simulink model "sim_validation_6DoFDQG_3DoF_fullq"  (R2024b)
settings: Solver=VariableStepAuto  StartTime=0.0  StopTime=tf  RelTol=1e-12  AbsTol=1e-12
values from neighbouring files (symbols this model uses):
  alpha = 0.5086    [3DoF_deterministic_Workspace.mat]    (also in Compressed_Time_Step_2dof_Experiment.mat; Copy_of_Deterministic_6DoF.m; Copy_of_Deterministic_6DoF_quat.m; Copy_of_SCP_Earth_Mars_transfer_GA_uniform_adaptive.m = 1)
  I = 0.15    [3DoF_deterministic_Workspace.mat]    (also in Copy_of_DQG_6DoF_fixedtf.m = [4.2; 4.2; 0.6]; Copy_of_Deterministic_6DoF.m = [50000; 150000; 150000] * (1e-3) ^ 2; Copy_of_Deterministic_6DoF_quat.m = [50000; 150000; 150000] * (1e-3) ^ 2; DQG_6DoF.m = [4.2; 4.2; 0.6])
  input_vector = 1:nu    [Deterministic_3DoF_with_mass_convexified_reynolds.m]    (also in Deterministic_3DoF_with_mass_convexified_takeoffdivert.m; Deterministic_3DoF_with_mass_polar.m; Deterministic_6DoF.m; Deterministic_6DoF_reynolds.m)
  L = 0.003    [3DoF_deterministic_Workspace.mat]    (also in Compressed_Time_Step_2dof_Experiment.mat; Copy_of_DQG_6DoF_fixedtf.m = 1; Copy_of_Deterministic_6DoF.m; Copy_of_Deterministic_6DoF_quat.m)
  m_0 = 2100    [3DoF_deterministic_Workspace.mat]    (also in Compressed_Time_Step_2dof_Experiment.mat = 2000; Copy_of_Deterministic_6DoF.m = 2600; Copy_of_Deterministic_6DoF_quat.m = 2600; Copy_of_SCP_Earth_Mars_transfer_GA_uniform_adaptive.m = 1)
  r_0_6DoF = [r_0(1); 0; r_0(2)]    [Deterministic_3DoF_with_mass_convexified_reynolds.m]    (also in Deterministic_3DoF_with_mass_convexified_takeoffdivert.m; Deterministic_6DoF.m = r_0; Deterministic_6DoF_reynolds.m = r_0; Deterministic_6DoF_reynolds_quat_alphabeta.m = r_0)
  rpy_0_6DoF = [0; theta_0; 0]    [Deterministic_3DoF_with_mass_convexified_reynolds.m]    (also in Deterministic_3DoF_with_mass_convexified_takeoffdivert.m; Deterministic_6DoF.m = dcm2angle(angle2dcm(theta1_0, theta2_0, theta3_0,"XYX"), "ZY; Deterministic_6DoF_reynolds.m = dcm2angle(angle2dcm(theta1_0, theta2_0, theta3_0,"XYX"), "ZY; Deterministic_6DoF_reynolds_quat_alphabeta.m = [theta_3; theta_1; theta_2])
  v_0_b_6DoF = [v_0_b(1); 0; v_0_b(2)]    [Deterministic_3DoF_with_mass_convexified_reynolds.m]    (also in Deterministic_3DoF_with_mass_convexified_takeoffdivert.m; Deterministic_6DoF.m = v_0_b; Deterministic_6DoF_reynolds.m = v_0_b; Deterministic_6DoF_reynolds_quat_alphabeta.m = quat_rot(q_conj(q_0), v_0))
  w_0_6DoF = [0; w_0; 0]    [Deterministic_3DoF_with_mass_convexified_reynolds.m]    (also in Deterministic_3DoF_with_mass_convexified_takeoffdivert.m; Deterministic_6DoF.m = w_0; Deterministic_6DoF_reynolds.m = w_0; Deterministic_6DoF_reynolds_quat_alphabeta.m = w_0)
undefined symbols (not defined in the file or in its folder): construct_dual_quat
libraries: sharedtransform x2, aerolibanim x1, simulink_extras x1
settings Model: Creator=thatf  LastModifiedBy=thatf

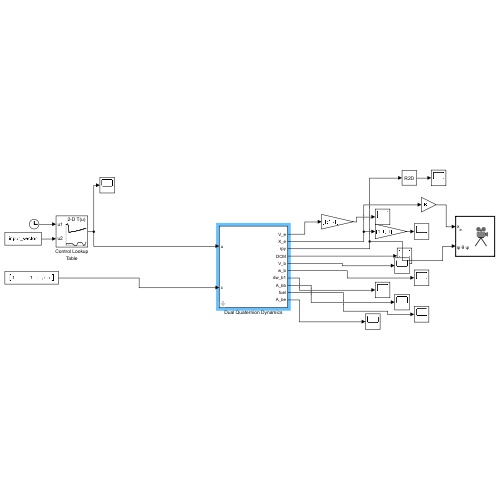
[thumbnail: Simulink's stored preview of the top-level diagram]
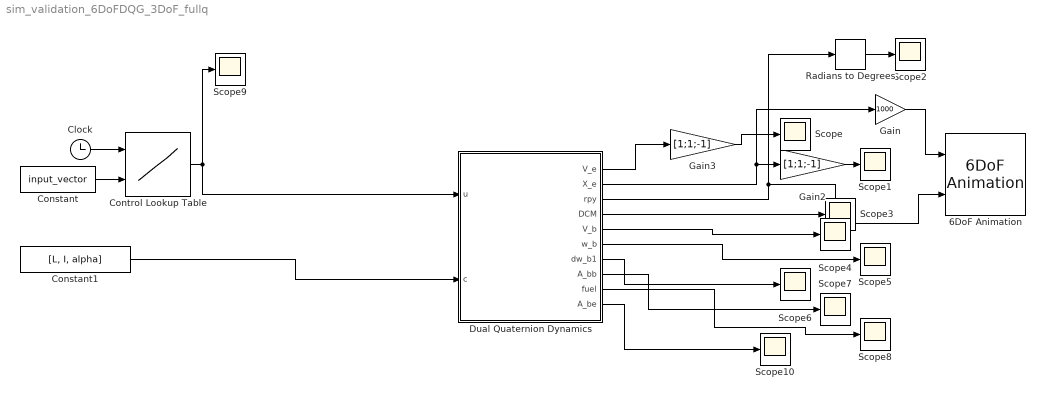
== system sim_validation_6DoFDQG_3DoF_fullq ==
  6DoF Animation : aerolibanim/6DoF Animation  u1=[-1000 1000 -100 100 -5000 50]  u2=0.05  u3=100  u4=[0 0 0]  u5=Fly alongside  u6=[0 1000 0]  u7=80  u8=on
  Clock : Clock
  Constant : Constant  Value=input_vector
  Constant1 : Constant  Value=[L, I, alpha]
  Control Lookup Table : Lookup_n-D  BreakpointsForDimension1=opt_time'  BreakpointsForDimension2=input_vector  Table=control_inputs'  InternalRulePriority=Speed  RndMeth=Simplest
      settings: InputPortMap=u0,u1
  Dual Quaternion Dynamics : Subsystem  mask{m_0=m_0, v_B_0=v_0_b_6DoF, q_0=[0 1 0 0; 0 0 1 0; 0 0 0 1; 1 0 0 0] * angle2quat(rpy_0_6DoF(1), rpy_0_6DoF(2), rpy_0_6DoF(3))', r_0=r_0_6DoF .* [1; 1; -1], w_B_0=w_0_6DoF}
      mask prompts: m_0 "Initial Mass"; v_B_0 "Initial Body Velocity"; q_0 "Initial Quaternion"; r_0 "Initial Position"; w_B_0 "Initial Body Angular Velocity"
  Gain : Gain  Gain=1000
  Gain2 : Gain  Gain=[1;1;-1]
  Gain3 : Gain  Gain=[1;1;-1]
  Radians to Degrees : simulink_extras/Transformations/Radians to Degrees
  Scope{,1..10} (11 alike) : Scope
  wires:
  Dual Quaternion Dynamics/3(rpy) -> 6DoF Animation/2, Radians to Degrees/1
  Dual Quaternion Dynamics/4(DCM) -> Scope3/1
  Dual Quaternion Dynamics/5(V_b) -> Scope4/1
  Dual Quaternion Dynamics/6(w_b) -> Scope5/1
  Dual Quaternion Dynamics/7(dw_b1) -> Scope6/1
  Dual Quaternion Dynamics/8(A_bb) -> Scope7/1
  Dual Quaternion Dynamics/9(fuel) -> Scope8/1
  Dual Quaternion Dynamics/2(X_e) -> Gain/1, Gain2/1
  Constant/1 -> Control Lookup Table/2
  Clock/1 -> Control Lookup Table/1
  Control Lookup Table/1 -> Dual Quaternion Dynamics/1(u), Scope9/1
  Dual Quaternion Dynamics/10(A_be) -> Scope10/1
  Gain/1 -> 6DoF Animation/1
  Radians to Degrees/1 -> Scope2/1
  Gain2/1 -> Scope1/1
  Dual Quaternion Dynamics/1(V_e) -> Gain3/1
  Gain3/1 -> Scope/1
  Constant1/1 -> Dual Quaternion Dynamics/2(c)

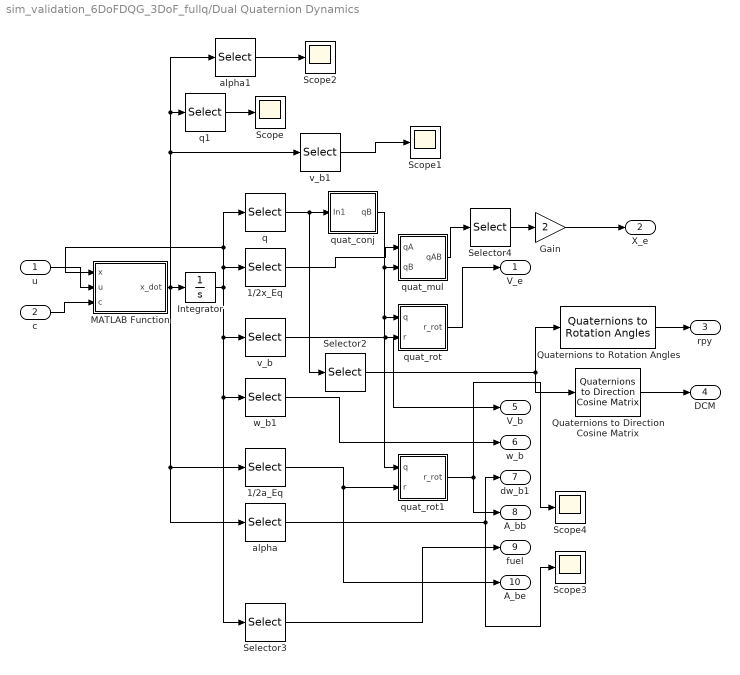
== system sim_validation_6DoFDQG_3DoF_fullq/Dual Quaternion Dynamics ==
  u : Inport
  c : Inport  Port=2
  1/2a_Eq : Selector  InputPortWidth=15  IndexOptions=Index vector (dialog)  Indices=[13:15]  OutputSizes=1
  1/2x_Eq : Selector  InputPortWidth=15  IndexOptions=Index vector (dialog)  Indices=[6:9]  OutputSizes=1
  Gain : Gain  Gain=2
  Integrator : Integrator  InitialCondition=[m_0; construct_dual_quat(q_0, r_0); w_B_0; v_B_0]
  MATLAB Function : MATLAB Function  TreatAsAtomicUnit=on
  Quaternions to Direction Cosine Matrix : sharedtransform/Quaternions to  Direction Cosine Matrix  aMode=aMode
      settings: LibrarySourceBlock=|
      | aerolibtransform2/Quaternions to
      | Direction Cosine Matrix
  Quaternions to Rotation Angles : sharedtransform/Quaternions to Rotation Angles  rotationOrder=ZYX  aMode=aMode
  Scope{,1..4} (5 alike) : Scope
  Selector2 : Selector  InputPortWidth=4  IndexOptions=Index vector (dialog)  Indices=[4 1 2 3]  OutputSizes=1
  Selector3 : Selector  InputPortWidth=15  IndexOptions=Index vector (dialog)  Indices=[1]  OutputSizes=1
  Selector4 : Selector  InputPortWidth=4  IndexOptions=Index vector (dialog)  Indices=[1:3]  OutputSizes=1
  alpha : Selector  InputPortWidth=15  IndexOptions=Index vector (dialog)  Indices=[10:12]  OutputSizes=1
  alpha1 : Selector  InputPortWidth=15  IndexOptions=Index vector (dialog)  Indices=[10:12]  OutputSizes=1
  q : Selector  InputPortWidth=15  IndexOptions=Index vector (dialog)  Indices=[2:5]  OutputSizes=1
  q1 : Selector  InputPortWidth=15  IndexOptions=Index vector (dialog)  Indices=[2:5]  OutputSizes=1
  quat_conj : Subsystem
  quat_mul : MATLAB Function  TreatAsAtomicUnit=on
  quat_rot : MATLAB Function  TreatAsAtomicUnit=on
  quat_rot1 : MATLAB Function  TreatAsAtomicUnit=on
  v_b : Selector  InputPortWidth=15  IndexOptions=Index vector (dialog)  Indices=[13:15]  OutputSizes=1
  v_b1 : Selector  InputPortWidth=15  IndexOptions=Index vector (dialog)  Indices=[13:15]  OutputSizes=1
  w_b1 : Selector  InputPortWidth=15  IndexOptions=Index vector (dialog)  Indices=[10:12]  OutputSizes=1
  V_e : Outport
  X_e : Outport  Port=2
  rpy : Outport  Port=3
  DCM : Outport  Port=4
  V_b : Outport  Port=5
  w_b : Outport  Port=6
  dw_b1 : Outport  Port=7
  A_bb : Outport  Port=8
  fuel : Outport  Port=9
  A_be : Outport  Port=10
  wires:
  u/1 -> MATLAB Function/2(u)
  c/1 -> MATLAB Function/3(c)
  MATLAB Function/1(x_dot) -> alpha1/1, q1/1, v_b1/1, alpha/1, 1/2a_Eq/1, Integrator/1
  Integrator/1 -> Selector3/1, w_b1/1, v_b/1, 1/2x_Eq/1, q/1, MATLAB Function/1(x)
  q/1 -> Selector2/1, quat_conj/1(In1)
  1/2x_Eq/1 -> quat_mul/1(qA)
  quat_conj/1(qB) -> quat_rot1/1(q), quat_rot/1(q), quat_mul/2(qB)
  quat_mul/1(qAB) -> Selector4/1
  v_b/1 -> quat_rot/2(r), V_b/1
  w_b1/1 -> w_b/1
  quat_rot/1(r_rot) -> V_e/1
  1/2a_Eq/1 -> quat_rot1/2(r), A_be/1
  quat_rot1/1(r_rot) -> A_bb/1, Scope4/1
  alpha/1 -> Scope3/1, dw_b1/1
  Selector2/1 -> Quaternions to Rotation Angles/1, Quaternions to Direction Cosine Matrix/1
  Quaternions to Rotation Angles/1 -> rpy/1
  Quaternions to Direction Cosine Matrix/1 -> DCM/1
  Selector3/1 -> fuel/1
  q1/1 -> Scope/1
  v_b1/1 -> Scope1/1
  alpha1/1 -> Scope2/1
  Selector4/1 -> Gain/1
  Gain/1 -> X_e/1

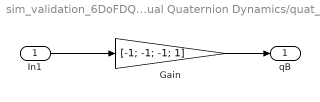
== system sim_validation_6DoFDQG_3DoF_fullq/Dual Quaternion Dynamics/quat_conj ==
  In1 : Inport
  Gain : Gain  Gain=[-1; -1; -1; 1]
  qB : Outport
  wires:
  In1/1 -> Gain/1
  Gain/1 -> qB/1

== matlab function sim_validation_6DoFDQG_3DoF_fullq/Dual Quaternion Dynamics/MATLAB Function ==
  data: x input; u input; x_dot output; c input
function x_dot = fcn(x, u, c)

m = x(1);
I = ones([3, 1]) * c(2);
L = c(1);
alpha = c(3);

qq = x(2:9);
q = x(2:5);
w_B = x(10:12);
v_B = x(13:15);
w = [w_B; v_B];

w_tilde = [w_B; 0; v_B; 0];

qq_dot = 1/2 * qq_mul(qq, w_tilde);

g_B = [0; 0; 0; quat_rot(q, [0; 0; 9.81e-3])]; % NEGATIVE BECAUSE Z IS DOWN

a_B = [u(1); 0; u(2)] .* [1; 1; -1]; % Z IS DOWN SO FLIP Z SIGN

J_mat = [zeros(3, 3), m * eye(3); diag(I), zeros(3, 3)];
J_inv = inv(J_mat);
Phi = [eye(3); skew([-L; 0; 0])];
w_dot = J_inv * (-qq_cross_matrix(w) * J_mat * w + Phi * a_B * m) + g_B;

m_dot = -alpha * norm(u(1:2)) * m;

x_dot = [m_dot; qq_dot; w_dot];

end

function qq_cross = qq_cross_matrix(qq)
    qq_cross = [skew(qq(1:3)), zeros(3, 3); skew(qq(4:6)), skew(qq(1:3))];
end

== matlab function sim_validation_6DoFDQG_3DoF_fullq/Dual Quaternion Dynamics/quat_mul ==
  data: qA input; qAB output; qB input
function qAB = fcn(qA, qB)

qAB = q_mul(qA, qB);

== matlab function sim_validation_6DoFDQG_3DoF_fullq/Dual Quaternion Dynamics/quat_rot ==
  data: q input; r_rot output; r input
function r_rot = fcn(q, r)

r_rot = quat_rot(q, r);

== matlab function sim_validation_6DoFDQG_3DoF_fullq/Dual Quaternion Dynamics/quat_rot1 ==
  data: q input; r_rot output; r input
function r_rot = fcn(q, r)

r_rot = quat_rot(q, r);
